simulink model "BeaconSearchSensor"  (R2018b)
settings: Solver=FixedStepDiscrete  StartTime=0.0  StopTime=inf  RelTol=1e-3
model workspace (MAT data in the model file):
  ForgetFactor = Simulink.Parameter
  ForgetFactor.Value = 0.9
  ForgetFactor.DataType = 'auto'
  ForgetFactor.Dimensions = [1 1]
  FundamentalFrequency = Simulink.Parameter
  FundamentalFrequency.Value = 40000
  FundamentalFrequency.DataType = 'auto'
  FundamentalFrequency.Dimensions = [1 1]
  Gain = Simulink.Parameter
  Gain.Value = 6
  Gain.DataType = 'auto'
  Gain.Dimensions = [1 1]
  TimeStep = Simulink.Parameter
  TimeStep.Value = 0.05
  TimeStep.DataType = 'auto'
  TimeStep.Dimensions = [1 1]
libraries: dspstat3 x2
settings Model: Creator=Apocalypse  LastModifiedBy=Apocalypse
settings OptimizationCC: DefaultParameterBehavior=Inlined  UseDivisionForNetSlopeComputation=on  UseFloatMulNetSlope=on  PassReuseOutputArgsAs=Individual arguments  ZeroExternalMemoryAtStartup=off  ZeroInternalMemoryAtStartup=off  NoFixptDivByZeroProtection=on  EfficientFloat2IntCast=on  LifeSpan=1  OptimizeBlockOrder=speed  DifferentSizesBufferReuse=on
settings DebuggingCC: ParameterTunabilityLossMsg=error
settings HardwareCC: ProdBitPerInt=16  ProdBitPerPointer=16  ProdBitPerSizeT=16  ProdBitPerPtrDiffT=16  ProdLargestAtomicFloat=None  ProdWordSize=8  ProdLongLongMode=on  ProdHWDeviceType=Atmel->AVR
settings SFSimCC: MATLABDynamicMemAlloc=off
settings RTWCC: SystemTargetFile=ert.tlc  GenCodeOnly=on  TemplateMakefile=ert_default_tmf  GenerateReport=on  BuildConfiguration=Faster Runs  IncludeHyperlinkInReport=on  LaunchReport=on  GenerateTraceInfo=on  GenerateTraceReport=on  GenerateTraceReportSl=on  GenerateTraceReportSf=on  GenerateTraceReportEml=on
settings RTWCC: CustomSourceCode=|
  | Servo BeaconSearchServo;
  | 
  | void GetBeaconLuminance(void)
  | {
  | 
  |     LeftBeaconLuminance = analogRead(LEFT_BEACON_SEARCH_SENSOR);
  |     //CenterBeaconLuminance = analogRead(CENTER_BEACON_SEARCH_SENSOR);
  |     RightBeaconLuminance = analogRead(RIGHT_BEACON_SEARCH_SENSOR);
  | }
  | 
  | void BeaconTrace(void)
  | {
  |     BeaconSearchServoAngle = BeaconSearchServoAngle + BeaconSearchSensorOutput;
  |     if(BeaconSearchServoAngle  < 0)
  |     {
  |         BeaconSearchServoAngle  = 0;
  |     }
  |     if(BeaconSearchServoAngle  >180)
  |     {
  |         BeaconSearchServoAngle  = 180;
  |     }
  |     BeaconSearchServo.write(BeaconSearchServoAngle);
  | }
settings RTWCC: CustomHeaderCode=|
  | #include <SPI.h>
  | #include <Servo.h>
  | extern const int LEFT_BEACON_SEARCH_SENSOR;
  | //extern const int CENTER_BEACON_SEARCH_SENSOR;
  | extern const int RIGHT_BEACON_SEARCH_SENSOR;
  | 
  | extern const int BEACON_SEARCH_SERVO_PIN;
  | extern volatile double BeaconSearchServoAngle;
  | 
  | extern void GetBeaconLuminance(void);
  | extern void BeaconTrace(void);
settings RTWCC: CustomInitializer=|
  | pinMode(LEFT_BEACON_SEARCH_SENSOR, INPUT);
  |   //pinMode(CENTER_BEACON_SEARCH_SENSOR, INPUT);
  |   pinMode(RIGHT_BEACON_SEARCH_SENSOR, INPUT);
  |   BeaconSearchServo.attach(BEACON_SEARCH_SERVO_PIN);
  |   BeaconSearchServo.write(90);
  |   BeaconSearchServoAngle = 90;
settings CodeAppCC: GenerateComments=off  IgnoreCustomStorageClasses=off  OperatorAnnotations=on  SimulinkDataObjDesc=on  SFDataObjDesc=on  CustomSymbolStrGlobalVar=rt$R$N$M  CustomSymbolStrType=$R$N$M  CustomSymbolStrFcn=$N$M$F  CustomSymbolStrMacro=$N$M  InsertBlockDesc=on
settings ERTTargetCC: TargetLangStandard=C99 (ISO)  CombineSignalStateStructs=on  SuppressErrorStatus=on  SupportComplex=off  InlinedParameterPlacement=NonHierarchical  RootIOFormat=Structure reference  ERTCustomFileTemplate=example_file_process.tlc  ERTFilePackagingFormat=Compact

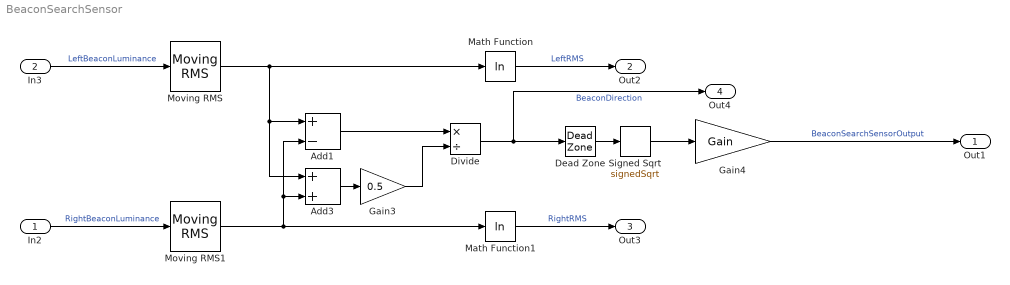
== system BeaconSearchSensor ==
  In2 : Inport
  In3 : Inport  Port=2
  Add1 : Sum  Inputs=+-
  Add3 : Sum
  Dead Zone : DeadZone  LowerValue=-0.01  UpperValue=0.01  SaturateOnIntegerOverflow=on
  Divide : Product  Inputs=*/
  Gain3 : Gain  Gain=0.5
  Gain4 : Gain  Gain=Gain
  Math Function : Math  Operator=log  SaturateOnIntegerOverflow=on
  Math Function1 : Math  Operator=log  SaturateOnIntegerOverflow=on
  Moving RMS : dspstat3/Moving RMS  Method=Exponential weighting  ForgettingFactorPort=off  SpecifyWindowLength=on  WindowLength=40  ForgettingFactor=ForgetFactor  SimulateUsing=Code generation
      settings: SourceProductName=DSP System Toolbox  SourceProductBaseCode=DS
  Moving RMS1 : dspstat3/Moving RMS  Method=Exponential weighting  ForgettingFactorPort=off  SpecifyWindowLength=on  WindowLength=40  ForgettingFactor=ForgetFactor  SimulateUsing=Code generation
      settings: SourceProductName=DSP System Toolbox  SourceProductBaseCode=DS
  Signed Sqrt : Sqrt  Operator=signedSqrt  SaturateOnIntegerOverflow=on
  Out1 : Outport
  Out2 : Outport  Port=2
  Out3 : Outport  Port=3
  Out4 : Outport  Port=4
  wires:
  In2/1 -> Moving RMS1/1  "RightBeaconLuminance"
  In3/1 -> Moving RMS/1  "LeftBeaconLuminance"
  Gain4/1 -> Out1/1  "BeaconSearchSensorOutput"
  Moving RMS/1 -> Math Function/1, Add3/1, Add1/1
  Moving RMS1/1 -> Math Function1/1, Add3/2, Add1/2
  Math Function/1 -> Out2/1  "LeftRMS"
  Math Function1/1 -> Out3/1  "RightRMS"
  Add3/1 -> Gain3/1
  Add1/1 -> Divide/1
  Gain3/1 -> Divide/2
  Divide/1 -> Out4/1, Dead Zone/1  "BeaconDirection"
  Signed Sqrt/1 -> Gain4/1
  Dead Zone/1 -> Signed Sqrt/1
